simulink model "lr41"  (R2022b)
settings: Solver=VariableStepAuto  StartTime=0.0  StopTime=200  MaxStep=0.01  MinStep=0.0001  RelTol=1e-3
InitFcn:
  | k0=6;
  | a0=-3;
  | a1=-4;
  | b0=2;
  | km0=12;
  | km1=36;
settings Model: Creator=thege  LastModifiedBy=Dimuss
settings DebuggingCC: UnconnectedInputMsg=warning  UnconnectedOutputMsg=warning  UnconnectedLineMsg=warning
settings ModelReferenceCC: EnableRefExpFcnMdlSchedulingChecks=on
settings RTWCC: DLArmComputeVersion=19.05

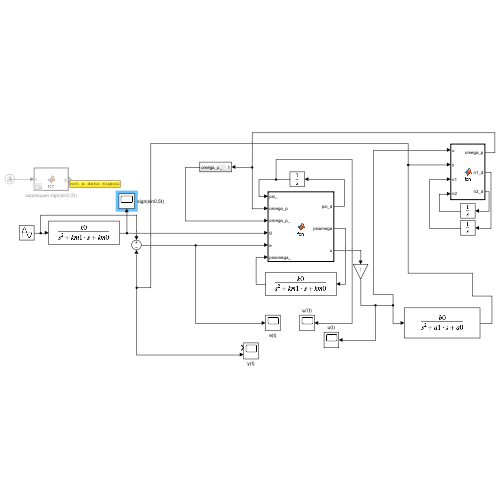
[thumbnail: Simulink's stored preview of the top-level diagram]
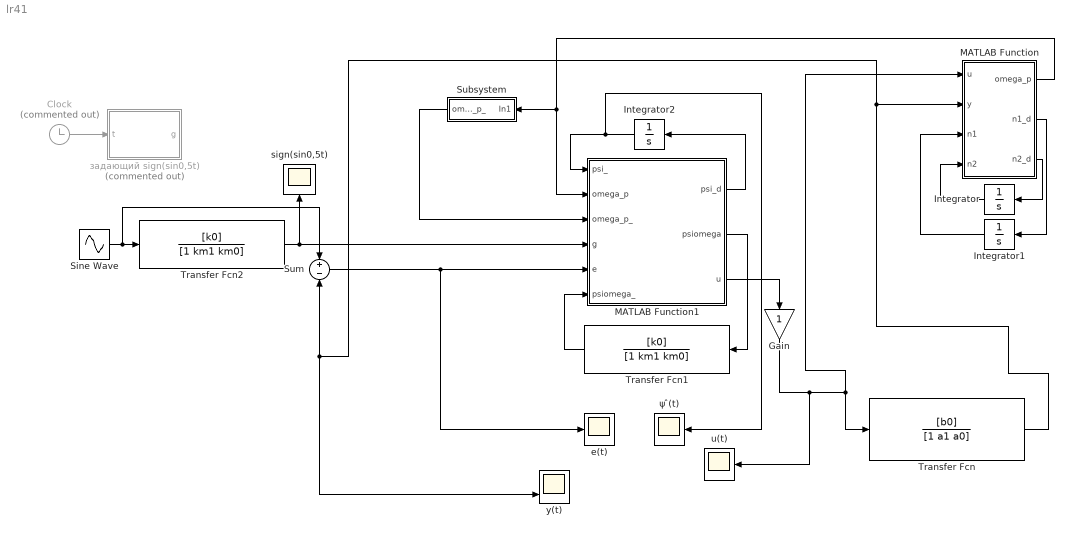
== system lr41 ==
  Clock : Clock  Commented=on
  Gain : Gain
  Integrator : Integrator
  Integrator1 : Integrator
  Integrator2 : Integrator  InitialCondition=[0 0 0]'
  MATLAB Function : MATLAB Function  TreatAsAtomicUnit=on
  MATLAB Function1 : MATLAB Function  TreatAsAtomicUnit=on
  Sine Wave : Sin  SampleTime=0
  Subsystem : Subsystem
  Sum : Sum  Inputs=+-
  Transfer Fcn : TransferFcn  Numerator=[b0]  Denominator=[1 a1 a0]
  Transfer Fcn1 : TransferFcn  Numerator=[k0]  Denominator=[1 km1 km0]
  Transfer Fcn2 : TransferFcn  Numerator=[k0]  Denominator=[1 km1 km0]
  e(t) : Scope
  sign(sin0,5t) : Scope
  u(t) : Scope
  y(t) : Scope  NumInputPorts=2
  ψ ̂(t) : Scope
  задающий sign(sin0,5t) : MATLAB Function  Commented=on  TreatAsAtomicUnit=on
  wires:
  Clock/1 -> задающий sign(sin0,5t)/1(t)
  Transfer Fcn/1 -> Sum/2, y(t)/2, MATLAB Function/2(y)
  Sum/1 -> e(t)/1, MATLAB Function1/5(e)
  MATLAB Function/3(n2_d) -> Integrator/1
  Integrator/1 -> MATLAB Function/4(n2)
  MATLAB Function/2(n1_d) -> Integrator1/1
  Integrator1/1 -> MATLAB Function/3(n1)
  MATLAB Function1/2(psiomega) -> Transfer Fcn1/1
  Transfer Fcn1/1 -> MATLAB Function1/6(psiomega_)
  Gain/1 -> u(t)/1, Transfer Fcn/1, MATLAB Function/1(u)
  MATLAB Function1/3(u) -> Gain/1
  MATLAB Function1/1(psi_d) -> Integrator2/1
  Integrator2/1 -> MATLAB Function1/1(psi_), ψ ̂(t)/1
  MATLAB Function/1(omega_p) -> MATLAB Function1/2(omega_p), Subsystem/1(In1)
  Subsystem/1(omega_p_) -> MATLAB Function1/3(omega_p_)
  Sine Wave/1 -> Sum/1, Transfer Fcn2/1
  Transfer Fcn2/1 -> sign(sin0,5t)/1, MATLAB Function1/4(g)

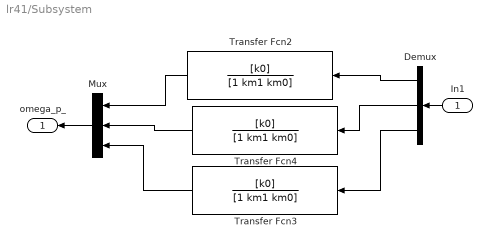
== system lr41/Subsystem ==
  In1 : Inport
  Demux : Demux  Outputs=3
  Mux : Mux  Inputs=3
  Transfer Fcn2 : TransferFcn  Numerator=[k0]  Denominator=[1 km1 km0]
  Transfer Fcn3 : TransferFcn  Numerator=[k0]  Denominator=[1 km1 km0]
  Transfer Fcn4 : TransferFcn  Numerator=[k0]  Denominator=[1 km1 km0]
  omega_p_ : Outport
  wires:
  Demux/2 -> Transfer Fcn4/1
  Demux/1 -> Transfer Fcn2/1
  Transfer Fcn4/1 -> Mux/2
  Demux/3 -> Transfer Fcn3/1
  Transfer Fcn2/1 -> Mux/1
  Mux/1 -> omega_p_/1
  In1/1 -> Demux/1
  Transfer Fcn3/1 -> Mux/3

== matlab function lr41/MATLAB Function1 ==
  data: psi_ input; psi_d output; psiomega output; omega_p input; omega_p_ input; g input; e input; psiomega_ input; u output; b0 parameter; k0 parameter
function [psi_d,psiomega,u]=fcn(psi_,omega_p,omega_p_,g,e,psiomega_, b0, k0)
psiomega=psi_'*omega_p;
e_=e-psi_'*omega_p_+psiomega_;
g1=0.1;
psi_d=g1*omega_p_*e_/(1+omega_p_'*omega_p_);
u=(psi_'*omega_p+k0*g)/b0;

== matlab function lr41/MATLAB Function ==
  data: u input; omega_p output; y input; n1 input; n2 input; n1_d output; n2_d output; k0 parameter
function [omega_p,n1_d,n2_d]=fcn(u,y,n1,n2, k0)
n1_d=-k0*n1+u;
n2_d=-k0*n2+y;
omega=[n1',n2',y]';
omega_p=-omega;

== matlab function lr41/задающий sign(sin0,5t) ==
  data: t input; g output
function g = fcn(t)
%g=2*sign(cos (t));
g = sign(sin(0.5*t));
